simulink model "model_DC_motor"  (Simulink 7.4)
settings: Solver=ode45  StartTime=0.0  StopTime=0.5  RelTol=1e-3
InitFcn:
  | clc;
  | clear;
  | 
  | %% Motor Data
  | Pn=25000;                       % Rated Poower of motor
  | Uan=400;                        % Rated voltage of motor
  | Ian=68;                         % Rated current of motor in ampere
  | Nn=1500;                        % Rated speed of motor in rpm
  | wn=(2*pi*Nn)/60;                % Converting rpm int rad/sec
  | J=0.16;                         % Inertia constant Nms^2
  | La=0.006;                       % Armature inductance 6mH
  | Tl=5;                           % Load torque
  | 
  | %% Calculating the resistance of motor
  | 
  | % Evaluating the flux
  | flux_e=(Pn/wn)/Ian;
  | 
  | % Evaluating the resistance
  | Ra=(Uan-wn*flux_e)/Ian;
StopFcn:
  | clc;
Description:
  | This file simulates the model of DC motor. It was developed by
  | 
  | Syed Abdul Rahman Kashif
  | UET Lahore/ UPB Germany
  | 
  | 05-01-2010
settings Model: Creator=Kashif  LastModifiedBy=Kashif

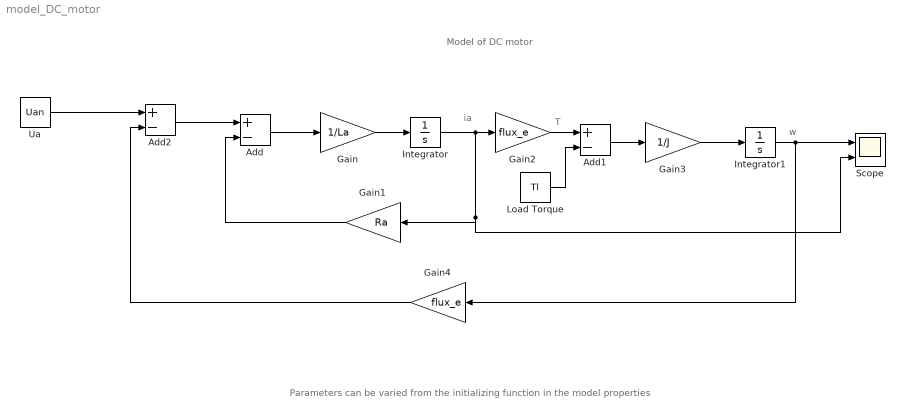
== system model_DC_motor ==
  note: ia
  note: T
  note: w
  note: Model of DC motor
  note: Parameters can be varied from the initializing function in the model properties
  Add : Sum  Inputs=+-  OutDataType=fixdt(1, 16)  OutScaling=2^-10
  Add1 : Sum  Inputs=+-  OutDataType=fixdt(1, 16)  OutScaling=2^-10
  Add2 : Sum  Inputs=+-  OutDataType=fixdt(1, 16)  OutScaling=2^-10
  Gain : Gain  Gain=1/La  ParameterDataType=fixdt(1, 16)  ParameterScaling=2^0  OutDataType=fixdt(1, 16)  OutScaling=2^0
  Gain1 : Gain  Gain=Ra  ParameterDataType=fixdt(1, 16)  ParameterScaling=2^0  OutDataType=fixdt(1, 16)  OutScaling=2^0
  Gain2 : Gain  Gain=flux_e  ParameterDataType=fixdt(1, 16)  ParameterScaling=2^0  OutDataType=fixdt(1, 16)  OutScaling=2^0
  Gain3 : Gain  Gain=1/J  ParameterDataType=fixdt(1, 16)  ParameterScaling=2^0  OutDataType=fixdt(1, 16)  OutScaling=2^0
  Gain4 : Gain  Gain=flux_e  ParameterDataType=fixdt(1, 16)  ParameterScaling=2^0  OutDataType=fixdt(1, 16)  OutScaling=2^0
  Integrator : Integrator
  Integrator1 : Integrator
  Load Torque : Constant  Value=Tl  OutDataType=fixdt(1, 16)  OutScaling=2^0
  Scope : Scope  NumInputPorts=2
      settings: YMin=-5~-5  YMax=5~5  MaxDataPoints=5000000
  Ua : Constant  Value=Uan  OutDataType=fixdt(1, 16)  OutScaling=2^0
  wires:
  Gain/1 -> Integrator/1
  Integrator/1 -> Gain2/1, Gain1/1, Scope/2
  Add/1 -> Gain/1
  Gain1/1 -> Add/2
  Gain2/1 -> Add1/1
  Add1/1 -> Gain3/1
  Gain3/1 -> Integrator1/1
  Add2/1 -> Add/1
  Gain4/1 -> Add2/2
  Integrator1/1 -> Gain4/1, Scope/1
  Load Torque/1 -> Add1/2
  Ua/1 -> Add2/1
